simulink model "Wiper_Project"  (R2023a)
settings: Solver=FixedStepDiscrete  StartTime=0.0  StopTime=20  FixedStep=0.01  RelTol=1e-3
libraries: simulink x1, SignalEditorBlockLib x1
settings Model: Creator=Alielden  LastModifiedBy=Alielden
settings OptimizationCC: DefaultParameterBehavior=Inlined  UseDivisionForNetSlopeComputation=on  GainParamInheritBuiltInType=on  UseFloatMulNetSlope=on  InlineInvariantSignals=on  PassReuseOutputArgsAs=Individual arguments  ZeroExternalMemoryAtStartup=off  ZeroInternalMemoryAtStartup=off  NoFixptDivByZeroProtection=on  EfficientFloat2IntCast=on  LifeSpan=1  OptimizeBlockOrder=speed  DifferentSizesBufferReuse=on  EfficientTunableParamExpr=on
settings DebuggingCC: ParameterTunabilityLossMsg=error
settings HardwareCC: ProdLongLongMode=on
settings SFSimCC: MATLABDynamicMemAlloc=off
settings RTWCC: Description=Embedded Coder  SystemTargetFile=ert.tlc  TemplateMakefile=ert_default_tmf
settings CodeAppCC: ForceParamTrailComments=on  IgnoreCustomStorageClasses=off  OperatorAnnotations=on  SimulinkDataObjDesc=on  SFDataObjDesc=on  CustomSymbolStrGlobalVar=rt$N$M  CustomSymbolStrType=$N$M  CustomSymbolStrFcn=$N$M$F  CustomSymbolStrMacro=$N$M  InsertBlockDesc=on
settings ERTTargetCC: TargetLangStandard=C99 (ISO)  GenerateSampleERTMain=on  IncludeMdlTerminateFcn=off  CombineSignalStateStructs=on  SupportComplex=off  SupportNonInlinedSFcns=on  InlinedParameterPlacement=NonHierarchical  ERTCustomFileTemplate=example_file_process.tlc  ERTFilePackagingFormat=CompactWithDataFile

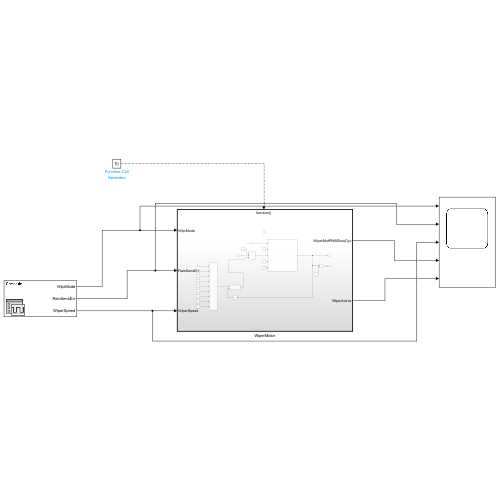
[thumbnail: Simulink's stored preview of the top-level diagram]
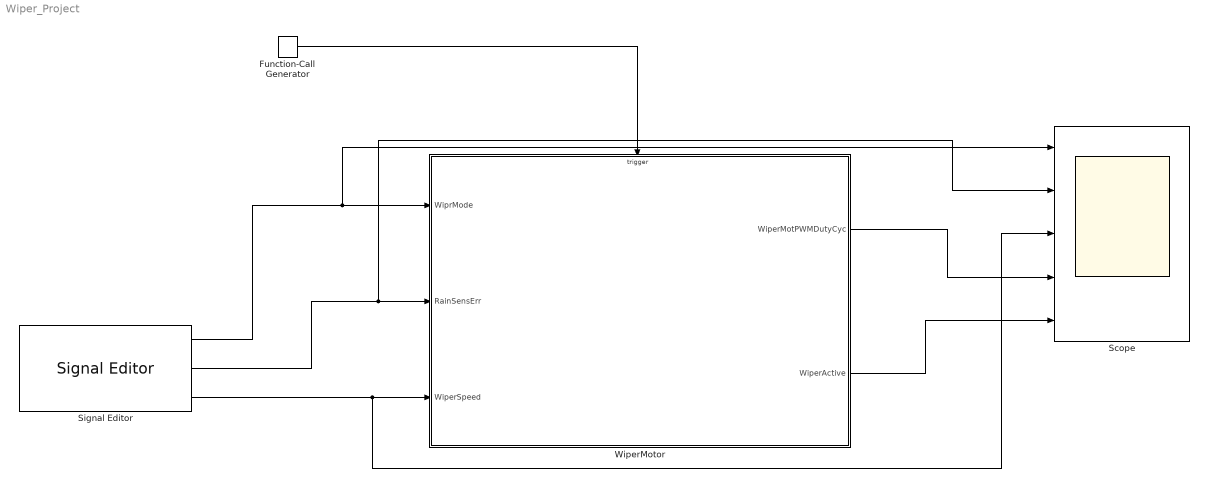
== system Wiper_Project ==
  Function-Call Generator : simulink/Ports & Subsystems/Function-Call Generator  sample_time=10e-3  numberOfIterations=1  DisallowWideOutput=off
  Scope : Scope  NumInputPorts=5
  Signal Editor : SignalEditorBlockLib/Signal Editor  FileName=D:\Model Based Design\Wiper_Project\Wiper_Project_Signal.mat  ActiveScenario=Scenario  ActiveSignal=WiprMode  IsBus=off  OutputBusObjectStr=Bus: BusObject  SampleTime=0  Interpolate=off  ZeroCross=off  OutputAfterFinalValue=Setting to zero  Unit=inherit  PreserveSignalName=on  ApplySigPropsToAllScenarios=on
  WiperMotor : Subsystem  TreatAsAtomicUnit=on
  wires:
  Function-Call Generator/1 -> WiperMotor/Trigger
  Signal Editor/2 -> Scope/2, WiperMotor/2(RainSensErr)
  Signal Editor/1 -> Scope/1, WiperMotor/1(WiprMode)
  WiperMotor/1(WiperMotPWMDutyCyc) -> Scope/4
  Signal Editor/3 -> Scope/3, WiperMotor/3(WiperSpeed)
  WiperMotor/2(WiperActive) -> Scope/5

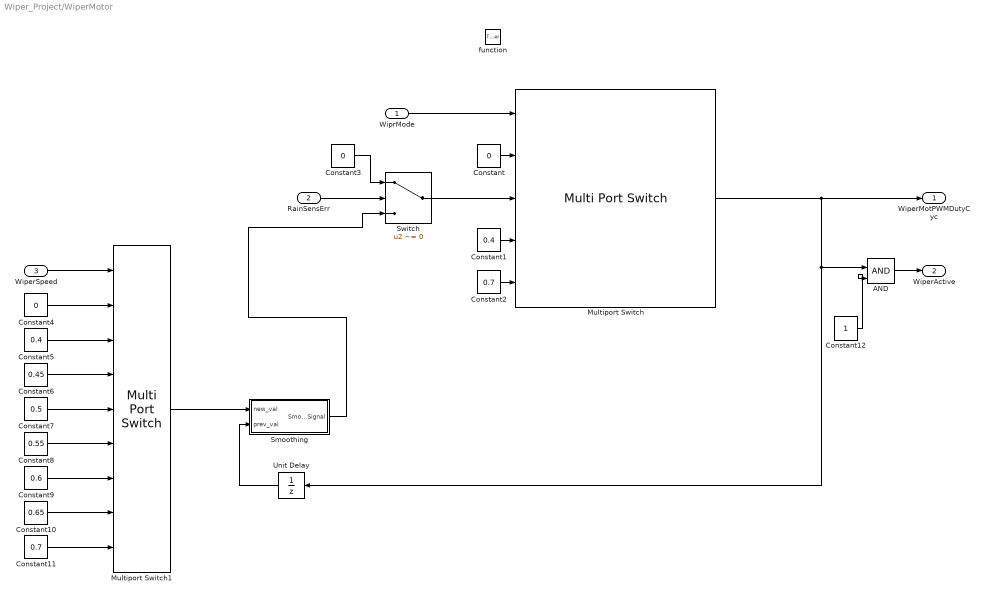
== system Wiper_Project/WiperMotor ==
  WiprMode : Inport
  RainSensErr : Inport  Port=2
  WiperSpeed : Inport  Port=3
  function : TriggerPort  TriggerType=function-call  VariantControl=(inherit)
  AND : Logic  IconShape=distinctive  AllPortsSameDT=off  OutDataTypeStr=boolean
  Constant : Constant  Value=0
  Constant1 : Constant  Value=0.4
  Constant10 : Constant  Value=0.65
  Constant11 : Constant  Value=0.7
  Constant12 : Constant
  Constant2 : Constant  Value=0.7
  Constant3 : Constant  Value=0
  Constant4 : Constant  Value=0
  Constant5 : Constant  Value=0.4
  Constant6 : Constant  Value=0.45
  Constant7 : Constant  Value=0.5
  Constant8 : Constant  Value=0.55
  Constant9 : Constant  Value=0.6
  Multiport Switch : MultiPortSwitch  DataPortOrder=Zero-based contiguous  Inputs=4  zeroidx=on  SaturateOnIntegerOverflow=off  InputSameDT=off
  Multiport Switch1 : MultiPortSwitch  DataPortOrder=Zero-based contiguous  Inputs=8  zeroidx=on  SaturateOnIntegerOverflow=off  InputSameDT=off
  Smoothing : Subsystem
  Switch : Switch  Criteria=u2 ~= 0  SaturateOnIntegerOverflow=off  InputSameDT=off
  Unit Delay : UnitDelay  SampleTime=-1  HasFrameUpgradeWarning=on
  WiperMotPWMDutyCyc : Outport
  WiperActive : Outport  Port=2
  wires:
  Constant11/1 -> Multiport Switch1/9
  Constant8/1 -> Multiport Switch1/6
  Constant9/1 -> Multiport Switch1/7
  Constant7/1 -> Multiport Switch1/5
  Smoothing/1(SmoothSignal) -> Switch/3
  Multiport Switch/1 -> AND/1, Unit Delay/1, WiperMotPWMDutyCyc/1
  WiprMode/1 -> Multiport Switch/1
  Switch/1 -> Multiport Switch/3
  Constant2/1 -> Multiport Switch/5
  Constant6/1 -> Multiport Switch1/4
  AND/1 -> WiperActive/1
  Constant10/1 -> Multiport Switch1/8
  Multiport Switch1/1 -> Smoothing/1(new_val)
  RainSensErr/1 -> Switch/2
  WiperSpeed/1 -> Multiport Switch1/1
  Constant5/1 -> Multiport Switch1/3
  Constant4/1 -> Multiport Switch1/2
  Constant1/1 -> Multiport Switch/4
  Constant12/1 -> AND/2
  Constant3/1 -> Switch/1
  Unit Delay/1 -> Smoothing/2(prev_val)
  Constant/1 -> Multiport Switch/2

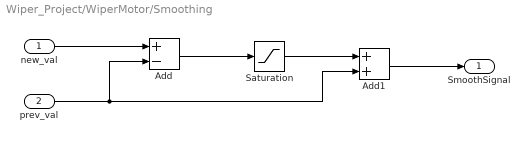
== system Wiper_Project/WiperMotor/Smoothing ==
  new_val : Inport
  prev_val : Inport  Port=2
  Add : Sum  Inputs=+-
  Add1 : Sum
  Saturation : Saturate  UpperLimit=0.005  LowerLimit=-0.005
  SmoothSignal : Outport
  wires:
  new_val/1 -> Add/1
  prev_val/1 -> Add1/2, Add/2
  Add/1 -> Saturation/1
  Saturation/1 -> Add1/1
  Add1/1 -> SmoothSignal/1
